simulink model "ModelKevin_Felipe_01"  (R2018a)
settings: Solver=ode45  StartTime=0.0  StopTime=100  MaxStep=1e-4  RelTol=1e-3
values from neighbouring files (symbols this model uses):
  Ap = 0.0007068    [variablesms.m]
  Awr = 0.0058    [variablesms.m]
  b = 0.0000000001    (= 1e-10)    [variablesms.m]
  cpg = 1006    [variablesms.m]
  cpv = 1873.3    [variablesms.m]
  dg = 1.23    [variablesms.m]
  dv = 14.71    [variablesms.m]
  F1 = 0.001    [variablesms.m]
  F2 = 0.001    [variablesms.m]
  h = 1000    [variablesms.m]
  J = 0.004    [variablesms.m]
  l = 0.06    [variablesms.m]
  lwr = 0.06    [variablesms.m]
  Patm = 101.325    [variablesms.m]
  r = 0.02    [variablesms.m]
  Rg = 0.287    [variablesms.m]
  rp = 0.015    [variablesms.m]
  Tcold = 300    [variablesms.m]
  Thot = 600    [variablesms.m]
  V1 = 0.001    [variablesms.m]
  V2 = 0.001    [variablesms.m]
  Xwr = 0.04    [variablesms.m]
undefined symbols (not defined in the file or in its folder): sigbuilder_block
libraries: simulink x1
settings Model: SimulationMode=accelerator  Creator=Osorio  LastModifiedBy=Pc
settings OptimizationCC: LifeSpan=inf
settings DebuggingCC: SFExecutionAtInitializationDiag=none
settings HardwareCC: ProdBitPerSizeT=32  ProdBitPerPtrDiffT=32  ProdWordSize=32  ProdHWDeviceType=Specified
settings CodeAppCC: StateflowObjectComments=on
settings SimscapeCC: SimscapeNormalizeSystem=off

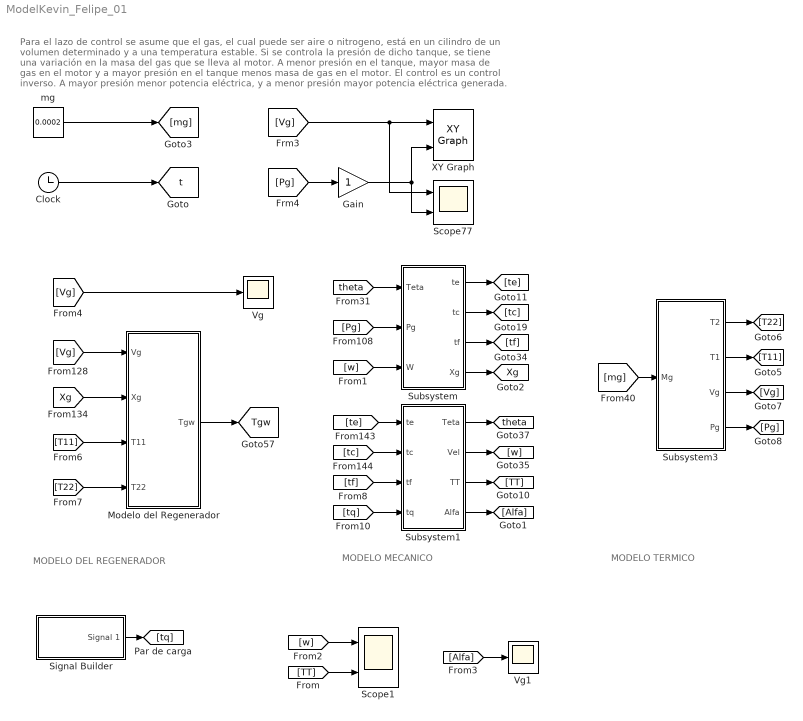
== system ModelKevin_Felipe_01 ==
  note: MODELO MECANICO
  note: Para el lazo de control se asume que el gas, el cual puede ser aire o nitrogeno, está en un cilindro de un volumen determinado y a una temperatura estable.
      | Si se controla la presión de dicho tanque, se tiene una variación en la masa del gas que se lleva al motor. A menor presión en el tanque, mayor masa de gas en el motor
      | y a mayor presión en el tanque menos masa de gas en el motor. El control es un control inverso. A mayor presión menor potencia eléctrica, y a menor presión
      | mayor potencia eléctrica generada.
  note: MODELO DEL REGENERADOR
  note: MODELO TERMICO
  Clock : Clock
  Gain : Gain
  Modelo del Regenerador : Subsystem
  Scope1 : Scope  NumInputPorts=2
  Scope77 : Scope  NumInputPorts=2
  Signal Builder : Subsystem  Tag=STV Subsys  LoadFcn=sigbuilder_block('load');  StartFcn=sigbuilder_block('start');  StopFcn=sigbuilder_block('stop');  ClipboardFcn=sigbuilder_block('clipboard');  mask(Sigbuilder block){tuvar=[0:10]}
      mask help: Simulink:masks:SigbuilderBlock_MD
      mask init:
      | if ~strcmp(get_param(bdroot(gcbh),'SimulationStatus'),'stopped') tuvar = sigbuilder_block('maskInit'); end
      settings: CopyFcn=sigbuilder_block('copy');  DeleteFcn=sigbuilder_block('delete');  ModelCloseFcn=sigbuilder_block('modelClose');  PreSaveFcn=sigbuilder_block('preSave');  PauseFcn=sigbuilder_block('pause');  ContinueFcn=sigbuilder_block('continue');  NameChangeFcn=sigbuilder_block('namechange');  OpenFcn=sigbuilder_block('open',[437.6 199.2 550.4 400 ]);  CloseFcn=sigbuilder_block('close');
      mask Display: plot(0, 0, 100, 100,[2, 2, 32, 32, 2], [68, 8, 8, 68, 68],[32, 2], [38, 38], [32, 19, 2],[53, 60, 44], [32, 17, 17, 2],[16, 16, 31, 31]);txt = getActiveGroup(gcbh);text(2, 100, txt,'verticalAlignment', 'top');
  Subsystem : Subsystem
  Subsystem1 : Subsystem
  Subsystem3 : Subsystem
  Vg : Scope
  Vg1 : Scope
  XY Graph : simulink/Sinks/XY Graph  xmin=0.00003  xmax=0.00009  ymin=0  ymax=2000  st=-1
  mg : Constant  Value=0.0002
  tag scope: Tgw=global, Xg=global, t=global, theta=global
  wires:
  Clock/1 -> [t]
  [Vg] -> Vg/1
  [Vg] -> Modelo del Regenerador/1(Vg)
  [Xg] -> Modelo del Regenerador/2(Xg)
  Modelo del Regenerador/1(Tgw) -> [Tgw]
  mg/1 -> [mg]
  [T11] -> Modelo del Regenerador/3(T11)
  [T22] -> Modelo del Regenerador/4(T22)
  [theta] -> Subsystem/1(Teta)
  [Pg] -> Subsystem/2(Pg)
  Subsystem/1(te) -> [te]
  Subsystem/2(tc) -> [tc]
  Subsystem/3(tf) -> [tf]
  Subsystem/4(Xg) -> [Xg]
  [tq] -> Subsystem1/4(tq)
  [te] -> Subsystem1/1(te)
  [tc] -> Subsystem1/2(tc)
  [tf] -> Subsystem1/3(tf)
  Subsystem1/1(Teta) -> [theta]
  Subsystem1/2(Vel) -> [w]
  Subsystem1/3(TT) -> [TT]
  Subsystem1/4(Alfa) -> [Alfa]
  [w] -> Subsystem/3(W)
  [mg] -> Subsystem3/1(Mg)
  Subsystem3/2(T1) -> [T11]
  Subsystem3/1(T2) -> [T22]
  Subsystem3/3(Vg) -> [Vg]
  [Vg] -> Scope77/1, XY Graph/1
  Subsystem3/4(Pg) -> [Pg]
  Signal Builder/1(Signal 1) -> [tq]
  [w] -> Scope1/1
  [TT] -> Scope1/2
  [Alfa] -> Vg1/1
  [Pg] -> Gain/1
  Gain/1 -> Scope77/2, XY Graph/2

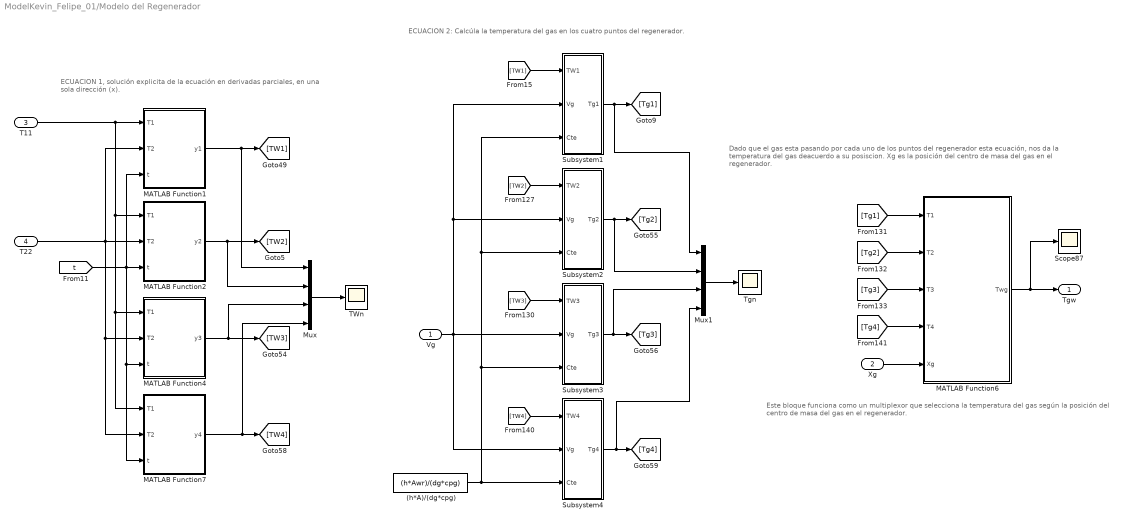
== system ModelKevin_Felipe_01/Modelo del Regenerador ==
  note: Este bloque funciona como un multiplexor que selecciona
      | la temperatura del gas según la posición del centro de masa del gas
      | en el regenerador.
  note: ECUACION 1, solución explicita de la ecuación en derivadas parciales,
      | en una sola dirección (x).
  note: ECUACION 2: Calcúla la temperatura del gas en los cuatro puntos del regenerador.
  note: Dado que el gas esta pasando por cada uno de los puntos del regenerador
      | esta ecuación, nos da la temperatura del gas deacuerdo a su posiscion.
      | Xg es la posición del centro de masa del gas en el regenerador.
  Vg : Inport
  Xg : Inport  Port=2
  T11 : Inport  Port=3
  T22 : Inport  Port=4
  (h*A)/(dg*cpg) : Constant  Value=(h*Awr)/(dg*cpg)
  MATLAB Function1 : MATLAB Function  TreatAsAtomicUnit=on
  MATLAB Function2 : MATLAB Function  TreatAsAtomicUnit=on
  MATLAB Function4 : MATLAB Function  TreatAsAtomicUnit=on
  MATLAB Function6 : MATLAB Function  TreatAsAtomicUnit=on
  MATLAB Function7 : MATLAB Function  TreatAsAtomicUnit=on
  Mux : Mux
  Mux1 : Mux
  Scope87 : Scope
  Subsystem1 : Subsystem
  Subsystem2 : Subsystem
  Subsystem3 : Subsystem
  Subsystem4 : Subsystem
  TWn : Scope
  Tgn : Scope
  Tgw : Outport
  wires:
  [t] -> MATLAB Function7/3(t), MATLAB Function4/3(t), MATLAB Function1/3(t), MATLAB Function2/3(t)
  Mux/1 -> TWn/1
  [TW4] -> Subsystem4/1(TW4)
  (h*A)/(dg*cpg)/1 -> Subsystem4/3(Cte), Subsystem3/3(Cte), Subsystem2/3(Cte), Subsystem1/3(Cte)
  [TW3] -> Subsystem3/1(TW3)
  Vg/1 -> Subsystem4/2(Vg), Subsystem3/2(Vg), Subsystem2/2(Vg), Subsystem1/2(Vg)
  MATLAB Function4/1(y3) -> Mux/3, [TW3]
  T11/1 -> MATLAB Function7/1(T1), MATLAB Function4/1(T1), MATLAB Function2/1(T1), MATLAB Function1/1(T1)
  MATLAB Function2/1(y2) -> Mux/2, [TW2]
  MATLAB Function7/1(y4) -> Mux/4, [TW4]
  MATLAB Function1/1(y1) -> Mux/1, [TW1]
  [TW1] -> Subsystem1/1(TW1)
  T22/1 -> MATLAB Function1/2(T2), MATLAB Function7/2(T2), MATLAB Function4/2(T2), MATLAB Function2/2(T2)
  [TW2] -> Subsystem2/1(TW2)
  Subsystem1/1(Tg1) -> Mux1/1, [Tg1]
  Subsystem4/1(Tg4) -> Mux1/4, [Tg4]
  Subsystem2/1(Tg2) -> Mux1/2, [Tg2]
  Subsystem3/1(Tg3) -> [Tg3], Mux1/3
  Mux1/1 -> Tgn/1
  [Tg4] -> MATLAB Function6/4(T4)
  [Tg3] -> MATLAB Function6/3(T3)
  [Tg1] -> MATLAB Function6/1(T1)
  MATLAB Function6/1(Twg) -> Tgw/1, Scope87/1
  [Tg2] -> MATLAB Function6/2(T2)
  Xg/1 -> MATLAB Function6/5(Xg)

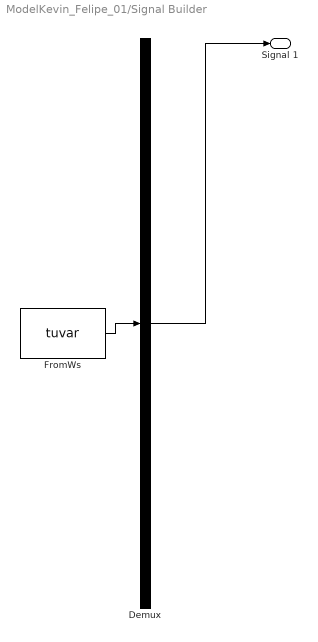
== system ModelKevin_Felipe_01/Signal Builder ==
  Demux : Demux  Tag=STV Demux  Outputs=1
  FromWs : FromWorkspace  Tag=STV FromWs  VariableName=tuvar  SampleTime=0
      SigBuilderData=|
      | common.afterFinalStr = 'Extrapolate'
      | common.sampleTime = 0
      | dataSet.timeRange = [0 50]
      | dataSet.name = 'Group 1'
      | sbobj.Groups.Name = 'Group 1'
      | sbobj.Groups.Signals.Name = 'Signal 1'
      | sbobj.Groups.Signals.XData = [0 50]
      | sbobj.Groups.Signals.YData = [0 0]
      | sbobj.Groups.TimeRange = [0 50]
  Signal 1 : Outport  Tag=STV Outport
  wires:
  Demux/1 -> Signal 1/1
  FromWs/1 -> Demux/1

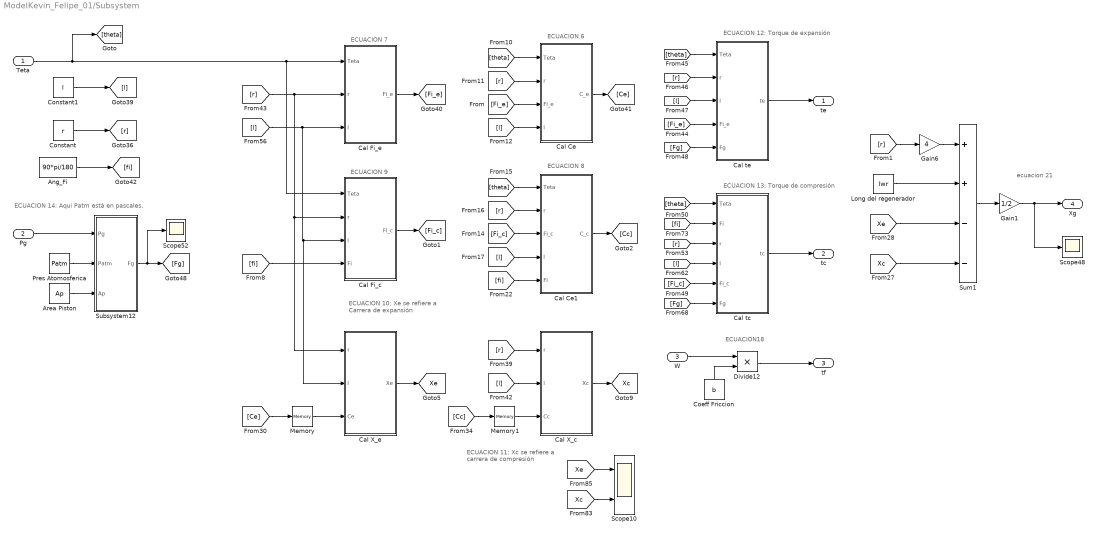
== system ModelKevin_Felipe_01/Subsystem ==
  note: ECUACION 11:
      | Xc se refiere a carrera de
      | compresión
  note: ECUACION 10:
      | Xe se refiere a Carrera de
      | expansión
  note: ECUACION 6
  note: ECUACION 7
  note: ECUACION18
  note: ECUACION 9
  note: ECUACION 8
  note: ECUACION 12: Torque de expansión
  note: ECUACION 13: Torque de compresión
  note: ECUACION 14: Aqui Patm está en pascales.
  note: ecuacion 21
  Teta : Inport
  Pg : Inport  Port=2
  W : Inport  Port=3
  Ang_Fi : Constant  Value=90*pi/180
  Area Piston : Constant  Value=Ap
  Cal Ce : MATLAB Function  TreatAsAtomicUnit=on
  Cal Ce1 : MATLAB Function  TreatAsAtomicUnit=on
  Cal Fi_c : MATLAB Function  TreatAsAtomicUnit=on
  Cal Fi_e : MATLAB Function  TreatAsAtomicUnit=on
  Cal X_c : MATLAB Function  TreatAsAtomicUnit=on
  Cal X_e : MATLAB Function  TreatAsAtomicUnit=on
  Cal tc : MATLAB Function  TreatAsAtomicUnit=on
  Cal te : MATLAB Function  TreatAsAtomicUnit=on
  Coeff Friccion : Constant  Value=b
  Constant : Constant  Value=r
  Constant1 : Constant  Value=l
  Divide12 : Product  Inputs=**
  Gain1 : Gain  Gain=1/2
  Gain6 : Gain  Gain=4
  Long del regenerador : Constant  Value=lwr
  Memory : Memory
  Memory1 : Memory
  Pres Atomosferica : Constant  Value=Patm
  Scope10 : Scope  NumInputPorts=2
  Scope48 : Scope
  Scope52 : Scope
  Subsystem12 : Subsystem
  Sum1 : Sum  Inputs=++--
  te : Outport
  tc : Outport  Port=2
  tf : Outport  Port=3
  Xg : Outport  Port=4
  tag scope: Xc=global, Xe=global
  wires:
  Cal tc/1(tc) -> tc/1
  [Fg] -> Cal tc/6(Fg)
  [l] -> Cal tc/4(l)
  [r] -> Cal tc/3(r)
  [theta] -> Cal tc/1(Teta)
  [Fi_c] -> Cal tc/5(Fi_c)
  [fi] -> Cal tc/2(Fi)
  Coeff Friccion/1 -> Divide12/2
  Divide12/1 -> tf/1
  Constant/1 -> [r]
  Constant1/1 -> [l]
  [Xe] -> Scope10/1
  W/1 -> Divide12/1
  [Xc] -> Scope10/2
  [r] -> Cal X_e/1(r), Cal Fi_c/2(r), Cal Fi_e/2(r)
  [fi] -> Cal Fi_c/4(Fi)
  [theta] -> Cal Ce/1(Teta)
  Teta/1 -> [theta], Cal Fi_c/1(Teta), Cal Fi_e/1(Teta)
  [r] -> Cal Ce/2(r)
  [l] -> Cal Ce/4(l)
  Ang_Fi/1 -> [fi]
  [l] -> Cal X_e/2(l), Cal Fi_c/3(l), Cal Fi_e/3(l)
  Cal Ce/1(C_e) -> [Ce]
  [Fi_e] -> Cal Ce/3(Fi_e)
  Cal Fi_c/1(Fi_c) -> [Fi_c]
  Cal Fi_e/1(Fi_e) -> [Fi_e]
  Cal X_e/1(Xe) -> [Xe]
  [r] -> Cal X_c/1(r)
  [Fi_c] -> Cal Ce1/3(Fi_c)
  [Ce] -> Memory/1
  [l] -> Cal X_c/2(l)
  [theta] -> Cal Ce1/1(Teta)
  [r] -> Cal Ce1/2(r)
  Cal X_c/1(Xc) -> [Xc]
  Cal Ce1/1(C_c) -> [Cc]
  [fi] -> Cal Ce1/5(Fi)
  [Cc] -> Memory1/1
  [l] -> Cal Ce1/4(l)
  Subsystem12/1(Fg) -> Scope52/1, [Fg]
  Area Piston/1 -> Subsystem12/3(Ap)
  Pg/1 -> Subsystem12/1(Pg)
  Pres Atomosferica/1 -> Subsystem12/2(Patm)
  [r] -> Cal te/2(r)
  [theta] -> Cal te/1(Teta)
  [Fg] -> Cal te/5(Fg)
  [Fi_e] -> Cal te/4(Fi_e)
  [l] -> Cal te/3(l)
  Cal te/1(te) -> te/1
  Long del regenerador/1 -> Sum1/2
  Gain6/1 -> Sum1/1
  [r] -> Gain6/1
  [Xe] -> Sum1/3
  [Xc] -> Sum1/4
  Sum1/1 -> Gain1/1
  Gain1/1 -> Xg/1, Scope48/1
  Memory/1 -> Cal X_e/3(Ce)
  Memory1/1 -> Cal X_c/3(Cc)

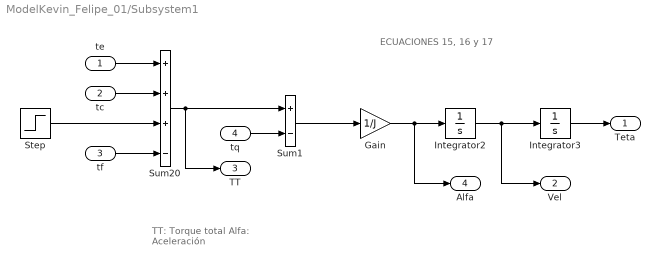
== system ModelKevin_Felipe_01/Subsystem1 ==
  note: TT: Torque total
      | Alfa: Aceleración
  note: ECUACIONES 15, 16 y 17
  te : Inport
  tc : Inport  Port=2
  tf : Inport  Port=3
  tq : Inport  Port=4
  Gain : Gain  Gain=1/J
  Integrator2 : Integrator  InitialCondition=1  AbsoluteTolerance=1
  Integrator3 : Integrator
  Step : Step  Time=2  Before=5  After=0
  Sum1 : Sum  Inputs=+-
  Sum20 : Sum  Inputs=+++-
  Teta : Outport
  Vel : Outport  Port=2
  TT : Outport  Port=3
  Alfa : Outport  Port=4
  wires:
  Sum20/1 -> TT/1, Sum1/1
  tc/1 -> Sum20/2
  te/1 -> Sum20/1
  Integrator2/1 -> Vel/1, Integrator3/1
  Integrator3/1 -> Teta/1
  Gain/1 -> Alfa/1, Integrator2/1
  tq/1 -> Sum1/2
  Sum1/1 -> Gain/1
  tf/1 -> Sum20/4
  Step/1 -> Sum20/3

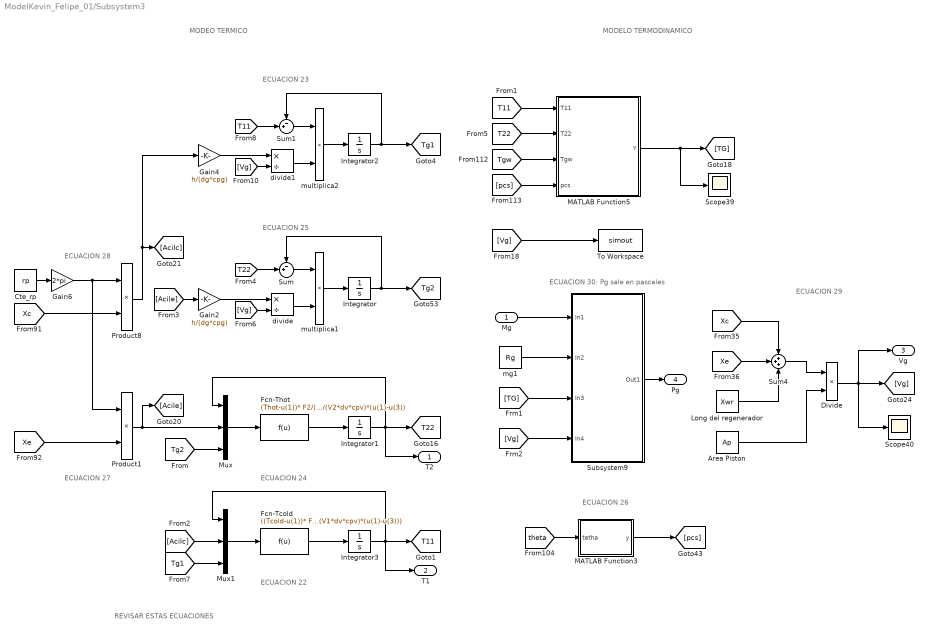
== system ModelKevin_Felipe_01/Subsystem3 ==
  note: REVISAR ESTAS ECUACIONES
  note: ECUACION 30: Pg sale en pascales
  note: ECUACION 27
  note: ECUACION 28
  note: ECUACION 24
  note: ECUACION 22
  note: MODELO TERMODINAMICO
  note: MODEO TERMICO
  note: ECUACION 26
  note: ECUACION 25
  note: ECUACION 23
  note: ECUACION 29
  Mg : Inport
  Area Piston : Constant  Value=Ap
  Cte_rp : Constant  Value=rp
  Divide : Product  Inputs=**
  Fcn-Tcold : Fcn  Expr=((Tcold-u(1))* F1/(V1*dv)-h*u(2)/(V1*dv*cpv)*(u(1)-u(3)))
  Fcn-Thot : Fcn  Expr=(Thot-u(1))* F2/(V2*dv)-h*u(2)/(V2*dv*cpv)*(u(1)-u(3))
  Gain2 : Gain  Gain=h/(dg*cpg)
  Gain4 : Gain  Gain=h/(dg*cpg)
  Gain6 : Gain  Gain=2*pi
  Integrator{,1..3} (4 alike) : Integrator
  Long del regenerador : Constant  Value=Xwr
  MATLAB Function3 : MATLAB Function  TreatAsAtomicUnit=on
  MATLAB Function5 : MATLAB Function  TreatAsAtomicUnit=on
  Mux : Mux  Inputs=3
  Mux1 : Mux  Inputs=3
  Product1 : Product
  Product8 : Product
  Scope39 : Scope
  Scope40 : Scope
  Subsystem9 : Subsystem
  Sum : Sum  Inputs=-+|
  Sum1 : Sum  Inputs=-+|
  Sum4 : Sum  Inputs=+++
  To Workspace : ToWorkspace  VariableName=simout  SaveFormat=Timeseries  SampleTime=-1
  divide : Product  Inputs=*/
  divide1 : Product  Inputs=*/
  mg1 : Constant  Value=Rg
  multiplica1 : Product  Inputs=**
  multiplica2 : Product  Inputs=**
  T2 : Outport
  T1 : Outport  Port=2
  Vg : Outport  Port=3
  Pg : Outport  Port=4
  tag scope: T11=global, T22=global, Tg1=global, Tg2=global
  wires:
  Subsystem9/1(Out1) -> Pg/1
  [Vg] -> Subsystem9/4(In4)
  [TG] -> Subsystem9/3(In3)
  mg1/1 -> Subsystem9/2(In2)
  [T11] -> MATLAB Function5/1(T11)
  MATLAB Function3/1(y) -> [pcs]
  [Vg] -> To Workspace/1
  [pcs] -> MATLAB Function5/4(pcs)
  [T22] -> MATLAB Function5/2(T22)
  MATLAB Function5/1(Y) -> Scope39/1, [TG]
  [Tgw] -> MATLAB Function5/3(Tgw)
  [theta] -> MATLAB Function3/1(tetha)
  Gain6/1 -> Product1/1, Product8/1
  Cte_rp/1 -> Gain6/1
  Product1/1 -> Mux/2, [Acile]
  [Xc] -> Product8/2
  [Xe] -> Product1/2
  multiplica1/1 -> Integrator/1
  Sum/1 -> multiplica1/1
  [T22] -> Sum/2
  Integrator/1 -> [Tg2], Sum/1
  Gain2/1 -> divide/1
  divide/1 -> multiplica1/2
  [Vg] -> divide/2
  Mux/1 -> Fcn-Thot/1
  Integrator1/1 -> T2/1, [T22], Mux/1
  Fcn-Thot/1 -> Integrator1/1
  [Tg2] -> Mux/3
  [Tg1] -> Mux1/3
  Fcn-Tcold/1 -> Integrator3/1
  Integrator3/1 -> T1/1, Mux1/1, [T11]
  Mux1/1 -> Fcn-Tcold/1
  [Vg] -> divide1/2
  divide1/1 -> multiplica2/2
  Gain4/1 -> divide1/1
  Integrator2/1 -> Sum1/1, [Tg1]
  [T11] -> Sum1/2
  Sum1/1 -> multiplica2/1
  multiplica2/1 -> Integrator2/1
  Product8/1 -> Gain4/1, [Acilc]
  Divide/1 -> Vg/1, [Vg], Scope40/1
  Mg/1 -> Subsystem9/1(In1)
  [Acilc] -> Mux1/2
  [Acile] -> Gain2/1
  [Xe] -> Sum4/2
  [Xc] -> Sum4/1
  Long del regenerador/1 -> Sum4/3
  Sum4/1 -> Divide/1
  Area Piston/1 -> Divide/2

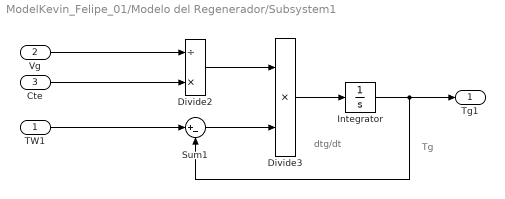
== system ModelKevin_Felipe_01/Modelo del Regenerador/Subsystem1 ==
  note: Tg
  note: dtg/dt
  TW1 : Inport
  Vg : Inport  Port=2
  Cte : Inport  Port=3
  Divide2 : Product  Inputs=/*
  Divide3 : Product  Inputs=**
  Integrator : Integrator
  Sum1 : Sum  Inputs=|+-
  Tg1 : Outport
  wires:
  Integrator/1 -> Sum1/2, Tg1/1
  TW1/1 -> Sum1/1
  Cte/1 -> Divide2/2
  Vg/1 -> Divide2/1
  Divide3/1 -> Integrator/1
  Divide2/1 -> Divide3/1
  Sum1/1 -> Divide3/2

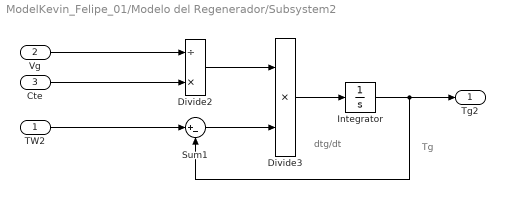
== system ModelKevin_Felipe_01/Modelo del Regenerador/Subsystem2 ==
  note: dtg/dt
  note: Tg
  TW2 : Inport
  Vg : Inport  Port=2
  Cte : Inport  Port=3
  Divide2 : Product  Inputs=/*
  Divide3 : Product  Inputs=**
  Integrator : Integrator
  Sum1 : Sum  Inputs=|+-
  Tg2 : Outport
  wires:
  Sum1/1 -> Divide3/2
  Divide2/1 -> Divide3/1
  Divide3/1 -> Integrator/1
  Vg/1 -> Divide2/1
  Cte/1 -> Divide2/2
  TW2/1 -> Sum1/1
  Integrator/1 -> Tg2/1, Sum1/2

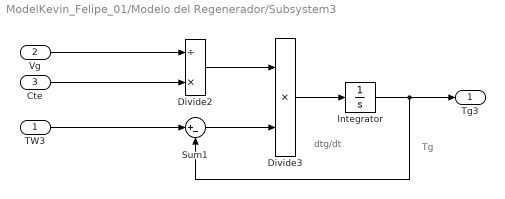
== system ModelKevin_Felipe_01/Modelo del Regenerador/Subsystem3 ==
  note: Tg
  note: dtg/dt
  TW3 : Inport
  Vg : Inport  Port=2
  Cte : Inport  Port=3
  Divide2 : Product  Inputs=/*
  Divide3 : Product  Inputs=**
  Integrator : Integrator
  Sum1 : Sum  Inputs=|+-
  Tg3 : Outport
  wires:
  Integrator/1 -> Sum1/2, Tg3/1
  TW3/1 -> Sum1/1
  Cte/1 -> Divide2/2
  Vg/1 -> Divide2/1
  Divide3/1 -> Integrator/1
  Divide2/1 -> Divide3/1
  Sum1/1 -> Divide3/2

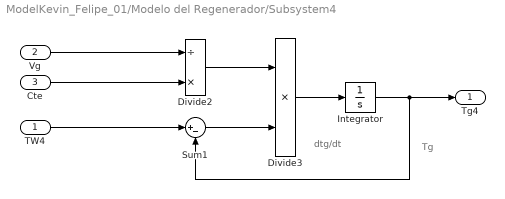
== system ModelKevin_Felipe_01/Modelo del Regenerador/Subsystem4 ==
  note: dtg/dt
  note: Tg
  TW4 : Inport
  Vg : Inport  Port=2
  Cte : Inport  Port=3
  Divide2 : Product  Inputs=/*
  Divide3 : Product  Inputs=**
  Integrator : Integrator
  Sum1 : Sum  Inputs=|+-
  Tg4 : Outport
  wires:
  Sum1/1 -> Divide3/2
  Divide2/1 -> Divide3/1
  Divide3/1 -> Integrator/1
  Vg/1 -> Divide2/1
  Cte/1 -> Divide2/2
  TW4/1 -> Sum1/1
  Integrator/1 -> Tg4/1, Sum1/2

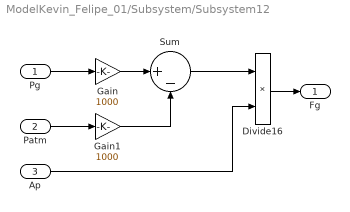
== system ModelKevin_Felipe_01/Subsystem/Subsystem12 ==
  Pg : Inport
  Patm : Inport  Port=2
  Ap : Inport  Port=3
  Divide16 : Product  Inputs=**
  Gain : Gain  Gain=1000
  Gain1 : Gain  Gain=1000
  Sum : Sum  Inputs=|+-
  Fg : Outport
  wires:
  Ap/1 -> Divide16/2
  Divide16/1 -> Fg/1
  Sum/1 -> Divide16/1
  Pg/1 -> Gain/1
  Patm/1 -> Gain1/1
  Gain/1 -> Sum/1
  Gain1/1 -> Sum/2

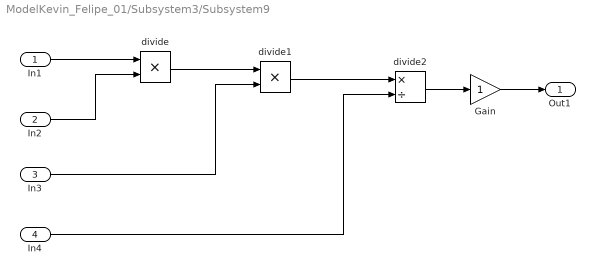
== system ModelKevin_Felipe_01/Subsystem3/Subsystem9 ==
  In1 : Inport
  In2 : Inport  Port=2
  In3 : Inport  Port=3
  In4 : Inport  Port=4
  Gain : Gain
  divide : Product  Inputs=**
  divide1 : Product  Inputs=**
  divide2 : Product  Inputs=*/
  Out1 : Outport
  wires:
  divide/1 -> divide1/1
  In3/1 -> divide1/2
  In1/1 -> divide/1
  In2/1 -> divide/2
  In4/1 -> divide2/2
  divide2/1 -> Gain/1
  divide1/1 -> divide2/1
  Gain/1 -> Out1/1

== matlab function ModelKevin_Felipe_01/Modelo del Regenerador/MATLAB Function1 ==
  data: T1 input; y1 output; T2 input; t input
function y1 = fcn(T1,T2,t)

% Initialize number of nodes and constants
N = 45;
ku = 15; % AISI 304 con ductividad termimica
rho = 7830; % AISI 304 densidad
cp = 500; % AISI 304 calor espe
L = 0.04;
q = 0;
h = L/(N-1); %delta de x
alfa=ku/(cp*rho);
dt = (0.5*(h^2))/alfa;
t = 20;
Ti = 300;
T0 = T2;
TL = T1;
r = (ku*dt)/(rho*cp*h^2);
if r>0.5
 error('disminuya el intervalo de tiempo dt')
end
% ubicaciÛn de los nodos
x = linspace(0,h,L);
% Temperatura incial en t = 0
jmax = round(t/dt);
u = zeros(N,jmax);
u(:,1) = Ti*ones(1,N);

u(1,:) = T0;
u(N,:) = TL;
for j = 1:jmax-1
 for i=2:N-1
 u(i,j+1) = (r*u(i-1,j)+(1-2*r)*u(i,j)+r*u(i+1,j)) + q*dt;
 end
end
%plot(u)
TW1=u(40,end);
y1=TW1;

== matlab function ModelKevin_Felipe_01/Subsystem3/MATLAB Function5 ==
  data: T11 input; Y output; T22 input; Tgw input; pcs input
function Y=fcn(T11,T22,Tgw,pcs)
u=0;
if pcs==1;
    u=Tgw;
end 

if pcs==2;
    u=T22;
end 

if pcs==3;
    u=Tgw;
end 

if pcs==4;
    u=T11;
end 

Y=u;

% pcs 1 calentamiento = Tgw
% pcs 2 expansion = Tge
% pcs 3 enfriamiento = Tgw
% pcs 4 compresion = Tgc

== matlab function ModelKevin_Felipe_01/Modelo del Regenerador/MATLAB Function2 ==
  data: T1 input; y2 output; T2 input; t input
function y2 = fcn(T1,T2,t)

% Initialize number of nodes and constants
N = 45;
ku = 15; % AISI 304 con ductividad termimica
rho = 7830; % AISI 304 densidad
cp = 500; % AISI 304 calor espe
L = 0.04;
q = 0;
h = L/(N-1); %delta de x
alfa=ku/(cp*rho);
dt = (0.5*(h^2))/alfa;
t = 20;
Ti = 300;
T0 = T2;
TL = T1;
r = (ku*dt)/(rho*cp*h^2);
if r>0.5
 error('disminuya el intervalo de tiempo dt')
end
% ubicaciÛn de los nodos
x = linspace(0,h,L);
% Temperatura incial en t = 0
jmax = round(t/dt);
u = zeros(N,jmax);
u(:,1) = Ti*ones(1,N);

u(1,:) = T0;
u(N,:) = TL;
for j = 1:jmax-1
 for i=2:N-1
 u(i,j+1) = (r*u(i-1,j)+(1-2*r)*u(i,j)+r*u(i+1,j)) + q*dt;
 end
end
%plot(u)
TW2=u(30,end);
y2=TW2;

== matlab function ModelKevin_Felipe_01/Subsystem3/MATLAB Function3 ==
  data: tetha input; y output
function y = fcn(tetha)


y=floor(4*((tetha/(2*3.1426))-floor(tetha/(2*3.1426))))+1;

== matlab function ModelKevin_Felipe_01/Modelo del Regenerador/MATLAB Function4 ==
  data: T1 input; y3 output; T2 input; t input
function y3 = fcn(T1,T2,t)

% Initialize number of nodes and constants
N = 45;
ku = 15; % AISI 304 con ductividad termimica
rho = 7830; % AISI 304 densidad
cp = 500; % AISI 304 calor espe
L = 0.04;
q = 0;
h = L/(N-1); %delta de x
alfa=ku/(cp*rho);
dt = (0.5*(h^2))/alfa;
t = 20;
Ti = 300;
T0 = T2;
TL = T1;
r = (ku*dt)/(rho*cp*h^2);
if r>0.5
 error('disminuya el intervalo de tiempo dt')
end
% ubicaciÛn de los nodos
x = linspace(0,h,L);
% Temperatura incial en t = 0
jmax = round(t/dt);
u = zeros(N,jmax);
u(:,1) = Ti*ones(1,N);

u(1,:) = T0;
u(N,:) = TL;
for j = 1:jmax-1
 for i=2:N-1
 u(i,j+1) = (r*u(i-1,j)+(1-2*r)*u(i,j)+r*u(i+1,j)) + q*dt;
 end
end
%plot(u)
TW3=u(20,end);

y3=TW3;

== matlab function ModelKevin_Felipe_01/Modelo del Regenerador/MATLAB Function6 ==
  data: T1 input; Twg output; T2 input; T3 input; T4 input; Xg input
function Twg = fcn(T1,T2,T3,T4,Xg)
u=0;
a=0.0337;
b=0.040;
c=0.0482;
d=0.0555;
e=0.0639;

if  (a<Xg) && (Xg<=b)
    
u=T1;
end

if (b<Xg) && (Xg<=c)
    
    u=T2;
end

if  (c<Xg) && (Xg<=d)
    
    u=T3;
end
if (d<Xg) && (Xg<=e)
    
    u=T4;
end

Twg=u;

== matlab function ModelKevin_Felipe_01/Modelo del Regenerador/MATLAB Function7 ==
  data: T1 input; y4 output; T2 input; t input
function y4 = fcn(T1,T2,t)

% Initialize number of nodes and constants
N = 45;
ku = 15; % AISI 304 con ductividad termimica
rho = 7830; % AISI 304 densidad
cp = 500; % AISI 304 calor espe
L = 0.04;
q = 0;
h = L/(N-1); %delta de x
alfa=ku/(cp*rho);
dt = (0.5*(h^2))/alfa;
t = 20;
Ti = 300;
T0 = T2;
TL = T1;
r = (ku*dt)/(rho*cp*h^2);
if r>0.5
 error('disminuya el intervalo de tiempo dt')
end
% ubicaciÛn de los nodos
x = linspace(0,h,L);
% Temperatura incial en t = 0
jmax = round(t/dt);
u = zeros(N,jmax);
u(:,1) = Ti*ones(1,N);

u(1,:) = T0;
u(N,:) = TL;
for j = 1:jmax-1
 for i=2:N-1
 u(i,j+1) = (r*u(i-1,j)+(1-2*r)*u(i,j)+r*u(i+1,j)) + q*dt;
 end
end
%plot(u)
TW4=u(1,end);

y4=TW4;

== matlab function ModelKevin_Felipe_01/Subsystem/Cal Fi_e ==
  data: Teta input; Fi_e output; r input; l input
function Fi_e = fcn(Teta,r,l)
Fi_e = asin(r*sin(Teta)/l);
end

== matlab function ModelKevin_Felipe_01/Subsystem/Cal Fi_c ==
  data: Teta input; Fi_c output; r input; l input; Fi input
function Fi_c = fcn(Teta,r,l,Fi)
Fi_c = asin(r*sin(Teta-Fi)/l);
end

== matlab function ModelKevin_Felipe_01/Subsystem/Cal Ce ==
  data: Teta input; C_e output; r input; Fi_e input; l input
function C_e = fcn(Teta,r,Fi_e,l)
C_e = r*cos(Teta)+l*cos(Fi_e);
end

== matlab function ModelKevin_Felipe_01/Subsystem/Cal Ce1 ==
  data: Teta input; C_c output; r input; Fi_c input; l input; Fi input
function C_c = fcn(Teta,r,Fi_c,l,Fi)
C_c = r*cos(Teta-Fi)+l*cos(Fi_c);
end

== matlab function ModelKevin_Felipe_01/Subsystem/Cal X_e ==
  data: r input; l input; Ce input; Xe output
function Xe = fcn(r,l,Ce)
Xe = r+l-Ce;
end

== matlab function ModelKevin_Felipe_01/Subsystem/Cal X_c ==
  data: r input; l input; Cc input; Xc output
function Xc = fcn(r,l,Cc)
Xc = r+l-Cc;
end

== matlab function ModelKevin_Felipe_01/Subsystem/Cal te ==
  data: Teta input; te output; r input; l input; Fi_e input; Fg input
function te = fcn(Teta,r,l,Fi_e,Fg)
te = Fg*tan(Fi_e)*(l-(r^2/(4*l))+r*cos(Teta)+r^2/(4*l)*cos(2*Teta));
end

== matlab function ModelKevin_Felipe_01/Subsystem/Cal tc ==
  data: Teta input; Fi input; tc output; r input; l input; Fi_c input; Fg input
function tc = fcn(Teta,Fi,r,l,Fi_c,Fg)
tc = Fg*tan(Fi_c)*(l-(r^2/(4*l))+r*cos(Teta-Fi)+r^2/(4*l)*cos(2*Teta-2*Fi));
end
